simulink model "System"  (R2020a)
settings: Solver=VariableStepAuto  StartTime=0.0  StopTime=10.0  RelTol=1e-3
values from neighbouring files (symbols this model uses):
  R = (r - T0')    [Control.m]
libraries: cstblocks x2
settings Model: Creator=Pim Ebbel de Bruin  LastModifiedBy=Pim Ebbel de Bruin

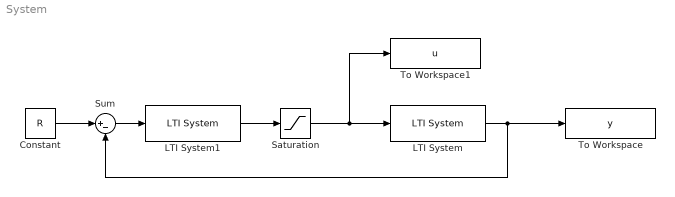
== system System ==
  Constant : Constant  Value=R
  LTI System : cstblocks/LTI System  sys=G  IC=[]
  LTI System1 : cstblocks/LTI System  sys=K  IC=[]
  Saturation : Saturate  UpperLimit=100  LowerLimit=0
  Sum : Sum  Inputs=|+-
  To Workspace : ToWorkspace  VariableName=y  SampleTime=-1
  To Workspace1 : ToWorkspace  VariableName=u  SampleTime=-1
  wires:
  LTI System/1 -> Sum/2, To Workspace/1
  Constant/1 -> Sum/1
  Sum/1 -> LTI System1/1
  LTI System1/1 -> Saturation/1
  Saturation/1 -> To Workspace1/1, LTI System/1
